simulink model "PubIfStateVSM_MDL"  (R2020b)
settings: configuration reference "DspaceConfig" (kept outside this file)
PostLoadFcn:
  | if any(exist('dsrtsu_mdlpostloadfcn', 'file') ~= 0), dsrtsu_mdlpostloadfcn('Execute', bdroot); end
InitFcn:
  | , if any(exist('rtifpga_mdlclblib', 'file') ~= 0), rtifpga_mdlclblib('Init', bdroot); end,
  | , if any(exist('dsmpb_private', 'file') ~= 0), dsmpb_private('dsmpb_mdlclblib', 'Init', bdroot); end,
model workspace (MAT data in the model file):
  P_VSM_ESS_DriverInputdSameDire_delaytime = Simulink.Parameter
  P_VSM_ESS_DriverInputdSameDire_delaytime.Value = 0.8
  P_VSM_ESS_DriverInputdSameDire_delaytime.DataType = 'single'
  P_VSM_ESS_DriverInputdSameDire_delaytime.Dimensions = [1 1]
  P_VSM_ESS_DrvOverTime_Paramsame = Simulink.Parameter
  P_VSM_ESS_DrvOverTime_Paramsame.Value = 1.2
  P_VSM_ESS_DrvOverTime_Paramsame.DataType = 'single'
  P_VSM_ESS_DrvOverTime_Paramsame.Dimensions = [1 1]
  P_VSM_PassSBRSpdIPLimt = Simulink.Parameter
  P_VSM_PassSBRSpdIPLimt.Value = 31
  P_VSM_PassSBRSpdIPLimt.DataType = 'uint8'
  P_VSM_PassSBRSpdIPLimt.Dimensions = [1 1]
  P_VSM_TJA_PassSBRSpdExistSlow = Simulink.Parameter
  P_VSM_TJA_PassSBRSpdExistSlow.Value = 30
  P_VSM_TJA_PassSBRSpdExistSlow.DataType = 'uint8'
  P_VSM_TJA_PassSBRSpdExistSlow.Dimensions = [1 1]
  User_ACCRes = Simulink.Signal
  User_ACCRes.DataType = 'auto'
  User_ACCRes.Dimensions = -1
  User_ACCRes.DimensionsMode = 'auto'
  User_ACCRes.Complexity = 'auto'
  User_ACCRes.SampleTime = -1
  User_ACCRes.SamplingMode = 'auto'
  User_ACCSet = Simulink.Signal
  User_ACCSet.DataType = 'auto'
  User_ACCSet.Dimensions = -1
  User_ACCSet.DimensionsMode = 'auto'
  User_ACCSet.Complexity = 'auto'
  User_ACCSet.SampleTime = -1
  User_ACCSet.SamplingMode = 'auto'
  User_TJASet = Simulink.Signal
  User_TJASet.DataType = 'auto'
  User_TJASet.Dimensions = -1
  User_TJASet.DimensionsMode = 'auto'
  User_TJASet.Complexity = 'auto'
  User_TJASet.SampleTime = -1
  User_TJASet.SamplingMode = 'auto'
PreSaveFcn:
  | , if any(exist('dsmpb_private', 'file') ~= 0), dsmpb_private('dsmpb_mdlclblib', 'PreSave', bdroot); end,
CloseFcn:
  | , if any(exist('dsmpb_private', 'file') ~= 0), dsmpb_private('dsmpb_mdlclblib', 'Close', bdroot); end,
settings Model: DataDictionary=HWA_DDs.sldd  RTICANMMDATA=struct('GeneralSetupData',struct('modelroot','D:\10_HWA_Project\Git_ADAS_Store\Adas\VSM_Test','generalsettings',struct('filesettings',struct('destfolder',struct('Name','RTICANMM_FILES','Check',1),'buildfolder',struct('Name','.','Check',1),'AbsDestfolder',struct('Name','D:\10_HWA_Project\Git_ADAS_Store\Adas\VSM_Test\RTICANMM_FILES'),'AbsBuildfolder',struct('Name','D:\10_HWA_Project\Git_ADAS_Store\Adas\VSM_Test'))),'options',struct('addpaths',1,'rmpaths',1,'addtrcexclusion',false,'cannavigator',struct('checkmonitoring',0),'show_usrtrc',0,'use_usrtrc',0),'advanced',struct('options',ones(1,100)),'MPSetup',{{}},'RTI',struct('Type','DSRT','Ver','4.4','Date','02-Nov-2020'),'modelname','PubIfStateVSM_MDL','block','PubIfStateVSM_MDL'))  DSRTSU_INTERNAL_RTIFPGA=170  Creator=GW00180895  LastModifiedBy=GW00201118
settings ConfigSetRef: SourceName=DspaceConfig

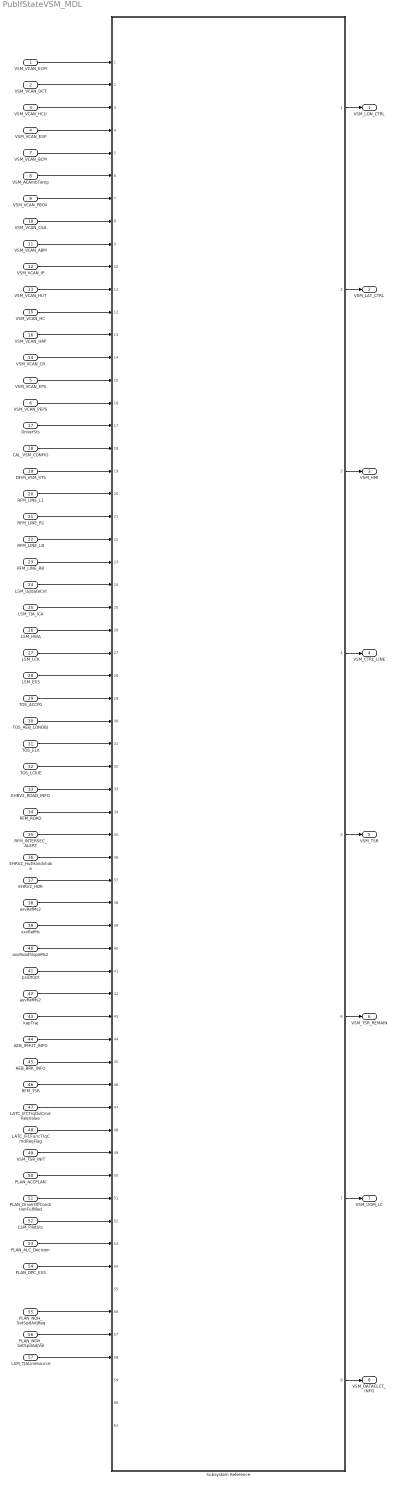
== system PubIfStateVSM_MDL ==
  VSM_VCAN_ECM : Inport  OutDataTypeStr=Bus: VCAN_ECM_MSG_BUS  PortDimensions=1  BusOutputAsStruct=on
  VSM_VCAN_DCT : Inport  Port=2  OutDataTypeStr=Bus: VCAN_DCT_MSG_BUS  PortDimensions=1  BusOutputAsStruct=on
  VSM_VCAN_HCU : Inport  Port=3  OutDataTypeStr=Bus: VCAN_HCU_MSG_BUS  PortDimensions=1  BusOutputAsStruct=on
  VSM_VCAN_ESP : Inport  Port=4  OutDataTypeStr=Bus: VCAN_ESP_MSG_BUS  PortDimensions=1  BusOutputAsStruct=on
  VSM_VCAN_EPS : Inport  Port=5  OutDataTypeStr=Bus: VCAN_EPS_MSG_BUS  PortDimensions=1  BusOutputAsStruct=on
  VSM_VCAN_PEPS : Inport  Port=6  OutDataTypeStr=Bus: VCAN_PEPS_MSG_BUS  PortDimensions=1  BusOutputAsStruct=on
  VSM_VCAN_BCM : Inport  Port=7  OutDataTypeStr=Bus: VCAN_BCM_MSG_BUS  PortDimensions=1  BusOutputAsStruct=on
  VSM_ACAmbTemp : Inport  Port=8  OutDataTypeStr=Bus: VCAN_AC_MSG_BUS  PortDimensions=1  BusOutputAsStruct=on
  VSM_VCAN_PBOX : Inport  Port=9  OutDataTypeStr=Bus: VCAN_PBOX_MSG_BUS  PortDimensions=1  BusOutputAsStruct=on
  VSM_VCAN_CSA : Inport  Port=10  OutDataTypeStr=Bus: VCAN_CSA_MSG_BUS  PortDimensions=1  BusOutputAsStruct=on
  VSM_VCAN_ABM : Inport  Port=11  OutDataTypeStr=Bus: VCAN_ABM_MSG_BUS  PortDimensions=1  BusOutputAsStruct=on
  VSM_VCAN_IP : Inport  Port=12  OutDataTypeStr=Bus: VCAN_IP_MSG_BUS  PortDimensions=1  BusOutputAsStruct=on
  VSM_VCAN_HUT : Inport  Port=13  OutDataTypeStr=Bus: VCAN_HUT_MSG_BUS  PortDimensions=1  BusOutputAsStruct=on
  VSM_VCAN_CR : Inport  Port=14  OutDataTypeStr=Bus: VCAN_CR_MSG_BUS  PortDimensions=1  BusOutputAsStruct=on
  VSM_VCAN_HC : Inport  Port=15  OutDataTypeStr=Bus: VCAN_HC_MSG_BUS  PortDimensions=1  BusOutputAsStruct=on
  VSM_VCAN_HAP : Inport  Port=16  OutDataTypeStr=Bus: VCAN_HAP_MSG_BUS  PortDimensions=1  BusOutputAsStruct=on
  DriverSts : Inport  Port=17  OutDataTypeStr=uint8  PortDimensions=1  BusOutputAsStruct=on
  CAL_VSM_CONFIG : Inport  Port=18  OutDataTypeStr=Bus: CAL_VSM_CONFIG_BUS  PortDimensions=1  BusOutputAsStruct=on
  DFIM_VSM_STS : Inport  Port=19  OutDataTypeStr=Bus: DFIM_VSM_STS_BUS  PortDimensions=1  BusOutputAsStruct=on
  RFM_LINE_L1 : Inport  Port=20  OutDataTypeStr=Bus: RFM_LINE_BUS  PortDimensions=1  BusOutputAsStruct=on
  RFM_LINE_R1 : Inport  Port=21  OutDataTypeStr=Bus: RFM_LINE_BUS  PortDimensions=1  BusOutputAsStruct=on
  RFM_LINE_LB : Inport  Port=22  OutDataTypeStr=Bus: RFM_LINE_BUS  PortDimensions=1  BusOutputAsStruct=on
  RFM_LINE_RB : Inport  Port=23  OutDataTypeStr=Bus: RFM_LINE_BUS  PortDimensions=1  BusOutputAsStruct=on
  LSM_UpdateCnt : Inport  Port=24  OutDataTypeStr=uint32  PortDimensions=1  BusOutputAsStruct=on
  LSM_TJA_ICA : Inport  Port=25  OutDataTypeStr=Bus: LSM_TJA_ICA_BUS  PortDimensions=1  BusOutputAsStruct=on
  LSM_HWA : Inport  Port=26  OutDataTypeStr=Bus: LSM_HWA_BUS  PortDimensions=1  BusOutputAsStruct=on
  LSM_LCK : Inport  Port=27  OutDataTypeStr=Bus: LSM_LCK_BUS  PortDimensions=1  BusOutputAsStruct=on
  LSM_ESS : Inport  Port=28  OutDataTypeStr=Bus: LSM_ESS_BUS  PortDimensions=1  BusOutputAsStruct=on
  TOS_ACCP0 : Inport  Port=29  OutDataTypeStr=Bus: TOS_ACCP0_BUS  PortDimensions=1  BusOutputAsStruct=on
  TOS_AEB_LONOBJ : Inport  Port=30  OutDataTypeStr=Bus: TOS_AEB_LONOBJ_BUS  PortDimensions=1  BusOutputAsStruct=on
  TOS_ELK : Inport  Port=31  OutDataTypeStr=Bus: TOS_ELK_BUS  PortDimensions=1  BusOutputAsStruct=on
  TOS_LCKIE : Inport  Port=32  OutDataTypeStr=Bus: TOS_LCKIE_BUS  PortDimensions=1  BusOutputAsStruct=on
  EHRV2_ROAD_INFO : Inport  Port=33  OutDataTypeStr=Bus: EHRV2_ROAD_INFO_BUS  PortDimensions=1  BusOutputAsStruct=on
  RFM_ROAD : Inport  Port=34  OutDataTypeStr=Bus: RFM_ROAD_BUS  PortDimensions=1  BusOutputAsStruct=on
  RFM_INTERSEC_ALERT : Inport  Port=35  OutDataTypeStr=Bus: RFM_INTERSEC_ALERT_BUS  PortDimensions=1  BusOutputAsStruct=on
  EHRV2_HutHandshake : Inport  Port=36  OutDataTypeStr=uint8  PortDimensions=1  BusOutputAsStruct=on
  EHRV2_HDR : Inport  Port=37  OutDataTypeStr=Bus: EHRV2_HDR_BUS  PortDimensions=1  BusOutputAsStruct=on
  axvRefMs2 : Inport  Port=38  OutDataTypeStr=single  PortDimensions=1  BusOutputAsStruct=on
  vxvRefMs : Inport  Port=39  OutDataTypeStr=single  PortDimensions=1  BusOutputAsStruct=on
  axvRoadSlopeMs2 : Inport  Port=40  OutDataTypeStr=single  PortDimensions=1  BusOutputAsStruct=on
  psiDtOpt : Inport  Port=41  OutDataTypeStr=single  PortDimensions=1  BusOutputAsStruct=on
  ayvRefMs2 : Inport  Port=42  OutDataTypeStr=single  PortDimensions=1  BusOutputAsStruct=on
  kapTraj : Inport  Port=43  OutDataTypeStr=single  PortDimensions=1  BusOutputAsStruct=on
  AEB_IPHUT_INFO : Inport  Port=44  OutDataTypeStr=Bus: AEB_IPHUT_INFO_BUS  PortDimensions=1  BusOutputAsStruct=on
  AEB_BRK_INFO : Inport  Port=45  OutDataTypeStr=Bus: AEB_BRK_INFO_BUS  PortDimensions=1  BusOutputAsStruct=on
  RFM_TSR : Inport  Port=46  OutDataTypeStr=Bus: RFM_TSR_BUS  PortDimensions=1  BusOutputAsStruct=on
  LATC_IFCTrqOvlCmdReqValue : Inport  Port=47  OutDataTypeStr=single  PortDimensions=1  BusOutputAsStruct=on
  LATC_IFCFuncTrqCmdReqFlag : Inport  Port=48  OutDataTypeStr=uint8  PortDimensions=1  BusOutputAsStruct=on
  VSM_TSR_INIT : Inport  Port=49  OutDataTypeStr=Bus: VSM_TSR_INIT_BUS  PortDimensions=1  BusOutputAsStruct=on
  PLAN_ACCPLAN : Inport  Port=50  OutDataTypeStr=Bus: PLAN_ACCPLAN_BUS  PortDimensions=1  BusOutputAsStruct=on
  PLAN_DriverOffConditionFulfilled : Inport  Port=51  OutDataTypeStr=boolean  PortDimensions=1  BusOutputAsStruct=on
  LSM_PilotSts : Inport  Port=52  OutDataTypeStr=uint8  PortDimensions=1  BusOutputAsStruct=on
  PLAN_ALC_Decision : Inport  Port=53  OutDataTypeStr=Bus: PLAN_ALC_DECS_BUS
  PLAN_DPC_ESS : Inport  Port=54  OutDataTypeStr=Bus: PLAN_DPC_ESS_BUS
  PLAN_NOH_SetSpdAdjReq : Inport  Port=55  OutDataTypeStr=boolean
  PLAN_NOH_SetSpdAdjVal : Inport  Port=56  OutDataTypeStr=uint8
  LSM_TJALineSource : Inport  Port=57
  Subsystem Reference : Subsystem  ReferencedSubsystem=PvtSubSys_VSM_ALL
  VSM_LON_CTRL : Outport  OutDataTypeStr=Bus: VSM_LON_CTRL_BUS  PortDimensions=1  BusOutputAsStruct=on
  VSM_LAT_CTRL : Outport  Port=2  OutDataTypeStr=Bus: VSM_LAT_CTRL_BUS  BusOutputAsStruct=on
  VSM_HMI : Outport  Port=3  OutDataTypeStr=Bus: VSM_HMI_BUS  PortDimensions=1  BusOutputAsStruct=on
  VSM_CTRL_LINE : Outport  Port=4  OutDataTypeStr=Bus: VSM_CTRL_LINE_BUS  PortDimensions=1  BusOutputAsStruct=on
  VSM_TSR : Outport  Port=5  OutDataTypeStr=Bus: VSM_TSR_BUS  PortDimensions=1  BusOutputAsStruct=on
  VSM_TSR_REMAIN : Outport  Port=6  OutDataTypeStr=Bus: VSM_TSR_REMAIN_BUS  BusOutputAsStruct=on
  VSM_UOM_LC : Outport  Port=7  OutDataTypeStr=Bus: VSM_UOM_LC_BUS  PortDimensions=1  BusOutputAsStruct=on
  VSM_DATACLCT_INFO : Outport  Port=8  OutDataTypeStr=Bus: VSM_DATACLCT_INFO_BUS  PortDimensions=1  BusOutputAsStruct=on
  wires:
  PLAN_ALC_Decision/1 -> Subsystem Reference/53
  VSM_VCAN_EPS/1 -> Subsystem Reference/15
  VSM_VCAN_CSA/1 -> Subsystem Reference/8
  RFM_LINE_RB/1 -> Subsystem Reference/23
  VSM_VCAN_IP/1 -> Subsystem Reference/10
  LSM_HWA/1 -> Subsystem Reference/26
  VSM_VCAN_HC/1 -> Subsystem Reference/12
  VSM_VCAN_HUT/1 -> Subsystem Reference/11
  EHRV2_ROAD_INFO/1 -> Subsystem Reference/33
  VSM_VCAN_PEPS/1 -> Subsystem Reference/16
  VSM_VCAN_HAP/1 -> Subsystem Reference/13
  axvRoadSlopeMs2/1 -> Subsystem Reference/40
  VSM_VCAN_ECM/1 -> Subsystem Reference/1
  VSM_VCAN_ABM/1 -> Subsystem Reference/9
  VSM_VCAN_PBOX/1 -> Subsystem Reference/7
  LSM_TJA_ICA/1 -> Subsystem Reference/25
  VSM_VCAN_CR/1 -> Subsystem Reference/14
  VSM_ACAmbTemp/1 -> Subsystem Reference/6
  EHRV2_HutHandshake/1 -> Subsystem Reference/36
  VSM_VCAN_BCM/1 -> Subsystem Reference/5
  RFM_TSR/1 -> Subsystem Reference/46
  Subsystem Reference/4 -> VSM_CTRL_LINE/1
  Subsystem Reference/8 -> VSM_DATACLCT_INFO/1
  LSM_PilotSts/1 -> Subsystem Reference/52
  Subsystem Reference/3 -> VSM_HMI/1
  Subsystem Reference/7 -> VSM_UOM_LC/1
  LATC_IFCTrqOvlCmdReqValue/1 -> Subsystem Reference/47
  Subsystem Reference/2 -> VSM_LAT_CTRL/1
  Subsystem Reference/6 -> VSM_TSR_REMAIN/1
  VSM_VCAN_HCU/1 -> Subsystem Reference/3
  Subsystem Reference/1 -> VSM_LON_CTRL/1
  Subsystem Reference/5 -> VSM_TSR/1
  PLAN_DriverOffConditionFulfilled/1 -> Subsystem Reference/51
  TOS_ELK/1 -> Subsystem Reference/31
  PLAN_NOH_SetSpdAdjVal/1 -> Subsystem Reference/57
  TOS_ACCP0/1 -> Subsystem Reference/29
  RFM_LINE_LB/1 -> Subsystem Reference/22
  CAL_VSM_CONFIG/1 -> Subsystem Reference/18
  PLAN_NOH_SetSpdAdjReq/1 -> Subsystem Reference/56
  TOS_AEB_LONOBJ/1 -> Subsystem Reference/30
  RFM_LINE_L1/1 -> Subsystem Reference/20
  PLAN_DPC_ESS/1 -> Subsystem Reference/54
  AEB_BRK_INFO/1 -> Subsystem Reference/45
  axvRefMs2/1 -> Subsystem Reference/38
  RFM_LINE_R1/1 -> Subsystem Reference/21
  VSM_VCAN_DCT/1 -> Subsystem Reference/2
  TOS_LCKIE/1 -> Subsystem Reference/32
  DFIM_VSM_STS/1 -> Subsystem Reference/19
  DriverSts/1 -> Subsystem Reference/17
  VSM_TSR_INIT/1 -> Subsystem Reference/49
  PLAN_ACCPLAN/1 -> Subsystem Reference/50
  LSM_UpdateCnt/1 -> Subsystem Reference/24
  LSM_ESS/1 -> Subsystem Reference/28
  VSM_VCAN_ESP/1 -> Subsystem Reference/4
  RFM_INTERSEC_ALERT/1 -> Subsystem Reference/35
  kapTraj/1 -> Subsystem Reference/43
  LSM_LCK/1 -> Subsystem Reference/27
  psiDtOpt/1 -> Subsystem Reference/41
  ayvRefMs2/1 -> Subsystem Reference/42
  RFM_ROAD/1 -> Subsystem Reference/34
  LATC_IFCFuncTrqCmdReqFlag/1 -> Subsystem Reference/48
  EHRV2_HDR/1 -> Subsystem Reference/37
  AEB_IPHUT_INFO/1 -> Subsystem Reference/44
  vxvRefMs/1 -> Subsystem Reference/39
  LSM_TJALineSource/1 -> Subsystem Reference/58
